simulink model "Task2A"  (R2019b)
settings: Solver=VariableStepAuto  StartTime=0.0  StopTime=10.0  MaxStep=1e-3  RelTol=1e-3
settings Model: Creator=sinow  LastModifiedBy=sinow

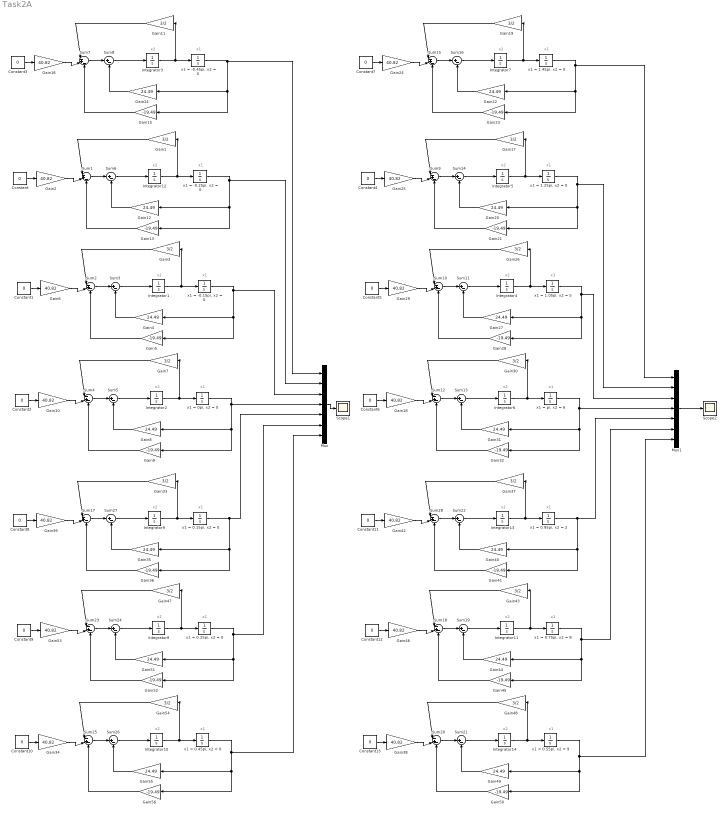
== system Task2A ==
  note: x1
  note: x2
  note: x2
  note: x1
  note: x2
  note: x1
  note: x2
  note: x1
  note: x1
  note: x2
  note: x1
  note: x2
  note: x2
  note: x1
  note: x1
  note: x2
  note: x1
  note: x2
  note: x1
  note: x2
  note: x1
  note: x2
  note: x2
  note: x1
  note: x1
  note: x1
  note: x2
  note: x2
  Constant{,1..13} (14 alike) : Constant  Value=0
  Gain{1,3,7,11,17,19,26,30,33,37,43,47..48,54} (14 alike) : Gain  Gain=3/2
  Gain{2,6,10,16,18,24..25,29,34,38..39,42,46,53} (14 alike) : Gain  Gain=40.82
  Gain{4,8,12,14,20,22,27,31,35,40,44,49,51,55} (14 alike) : Gain  Gain=24.49
  Gain{5,9,13,15,21,23,28,32,36,41,45,50,52,56} (14 alike) : Gain  Gain=-19.49
  Integrator{1..14} (14 alike) : Integrator
  Mux : Mux  Inputs=7
  Mux1 : Mux  Inputs=7
  Scope1 : Scope
  Scope2 : Scope
  Sum{1..2,4,7,9..10,12,15,17..18,20,23,25,28} (14 alike) : Sum  Inputs=|-+-
  Sum{3,5..6,8,11,13..14,16,19,21..22,24,26..27} (14 alike) : Sum  Inputs=|+-
  "x1 = -0.15pi, x2 = 0" : Integrator  InitialCondition=-0.15*pi
  "x1 = -0.25pi, x2 = 0" : Integrator  InitialCondition=-0.25*pi
  "x1 = -0.45pi, x2 = 0" : Integrator  InitialCondition=-0.45*pi
  "x1 = 0.15pi, x2 = 0" : Integrator  InitialCondition=0.15*pi
  "x1 = 0.25pi, x2 = 0" : Integrator  InitialCondition=0.25*pi
  "x1 = 0.45pi, x2 = 0" : Integrator  InitialCondition=0.45*pi
  "x1 = 0.55pi, x2 = 9" : Integrator  InitialCondition=0.55*pi
  "x1 = 0.75pi, x2 = 8" : Integrator  InitialCondition=0.75*pi
  "x1 = 0.95pi, x2 = 2" : Integrator  InitialCondition=0.95*pi
  "x1 = 0pi, x2 = 0" : Integrator
  "x1 = 1.05pi, x2 = 5" : Integrator  InitialCondition=1.05*pi
  "x1 = 1.25pi, x2 = 0" : Integrator  InitialCondition=1.25*pi
  "x1 = 1.45pi, x2 = 0" : Integrator  InitialCondition=1.45*pi
  "x1 = pi, x2 = 6" : Integrator  InitialCondition=pi
  wires:
  Gain13/1 -> Sum1/3
  Integrator12/1 -> Gain1/1, "x1 = -0.25pi, x2 = 0"/1
  Sum6/1 -> Integrator12/1
  Gain12/1 -> Sum6/2
  Gain1/1 -> Sum1/1
  Sum1/1 -> Sum6/1
  Gain2/1 -> Sum1/2
  Constant/1 -> Gain2/1
  Gain5/1 -> Sum2/3
  Sum3/1 -> Integrator1/1
  Integrator1/1 -> Gain3/1, "x1 = -0.15pi, x2 = 0"/1
  Gain4/1 -> Sum3/2
  Gain3/1 -> Sum2/1
  Constant1/1 -> Gain6/1
  Sum2/1 -> Sum3/1
  Gain6/1 -> Sum2/2
  "x1 = 0pi, x2 = 0"/1 -> Mux/4, Gain8/1, Gain9/1
  Gain9/1 -> Sum4/3
  Sum5/1 -> Integrator2/1
  Integrator2/1 -> Gain7/1, "x1 = 0pi, x2 = 0"/1
  Gain8/1 -> Sum5/2
  Gain7/1 -> Sum4/1
  Constant2/1 -> Gain10/1
  Sum4/1 -> Sum5/1
  Gain10/1 -> Sum4/2
  Gain15/1 -> Sum7/3
  Sum8/1 -> Integrator3/1
  Integrator3/1 -> Gain11/1, "x1 = -0.45pi, x2 = 0"/1
  Gain14/1 -> Sum8/2
  Gain11/1 -> Sum7/1
  Constant3/1 -> Gain16/1
  Sum7/1 -> Sum8/1
  Gain16/1 -> Sum7/2
  Sum14/1 -> Integrator5/1
  Integrator5/1 -> Gain17/1, "x1 = 1.25pi, x2 = 0"/1
  Gain20/1 -> Sum14/2
  Gain17/1 -> Sum9/1
  Sum12/1 -> Sum13/1
  Gain30/1 -> Sum12/1
  Constant6/1 -> Gain18/1
  Gain31/1 -> Sum13/2
  Gain18/1 -> Sum12/2
  Gain32/1 -> Sum12/3
  Sum10/1 -> Sum11/1
  Constant5/1 -> Gain29/1
  Integrator4/1 -> Gain26/1, "x1 = 1.05pi, x2 = 5"/1
  Sum11/1 -> Integrator4/1
  Gain25/1 -> Sum9/2
  Sum9/1 -> Sum14/1
  Gain26/1 -> Sum10/1
  Sum16/1 -> Integrator7/1
  Gain24/1 -> Sum15/2
  Integrator6/1 -> Gain30/1, "x1 = pi, x2 = 6"/1
  Gain22/1 -> Sum16/2
  Constant7/1 -> Gain24/1
  Gain19/1 -> Sum15/1
  Integrator7/1 -> Gain19/1, "x1 = 1.45pi, x2 = 0"/1
  Constant4/1 -> Gain25/1
  Sum15/1 -> Sum16/1
  Gain27/1 -> Sum11/2
  Sum13/1 -> Integrator6/1
  Gain29/1 -> Sum10/2
  Gain23/1 -> Sum15/3
  Gain28/1 -> Sum10/3
  Gain21/1 -> Sum9/3
  Gain36/1 -> Sum17/3
  Sum27/1 -> Integrator9/1
  Integrator9/1 -> Gain33/1, "x1 = 0.15pi, x2 = 0"/1
  Gain35/1 -> Sum27/2
  Gain33/1 -> Sum17/1
  Gain45/1 -> Sum18/3
  Gain41/1 -> Sum28/3
  Gain44/1 -> Sum19/2
  Constant11/1 -> Gain42/1
  Sum28/1 -> Sum22/1
  Gain43/1 -> Sum18/1
  Integrator11/1 -> Gain43/1, "x1 = 0.75pi, x2 = 8"/1
  Constant12/1 -> Gain46/1
  Sum18/1 -> Sum19/1
  Gain50/1 -> Sum20/3
  Integrator14/1 -> Gain48/1, "x1 = 0.55pi, x2 = 9"/1
  Gain40/1 -> Sum22/2
  Gain38/1 -> Sum20/2
  Gain48/1 -> Sum20/1
  Sum20/1 -> Sum21/1
  Gain49/1 -> Sum21/2
  Integrator13/1 -> Gain37/1, "x1 = 0.95pi, x2 = 2"/1
  Sum25/1 -> Sum26/1
  Sum21/1 -> Integrator14/1
  Gain54/1 -> Sum25/1
  Constant10/1 -> Gain34/1
  Gain55/1 -> Sum26/2
  Gain34/1 -> Sum25/2
  Gain56/1 -> Sum25/3
  Integrator10/1 -> Gain54/1, "x1 = 0.45pi, x2 = 0"/1
  Gain37/1 -> Sum28/1
  Sum26/1 -> Integrator10/1
  Gain46/1 -> Sum18/2
  Gain53/1 -> Sum23/2
  Sum23/1 -> Sum24/1
  Constant9/1 -> Gain53/1
  Integrator8/1 -> Gain47/1, "x1 = 0.25pi, x2 = 0"/1
  Gain52/1 -> Sum23/3
  Sum19/1 -> Integrator11/1
  Sum24/1 -> Integrator8/1
  Gain42/1 -> Sum28/2
  Gain51/1 -> Sum24/2
  Constant13/1 -> Gain38/1
  Sum22/1 -> Integrator13/1
  Constant8/1 -> Gain39/1
  Sum17/1 -> Sum27/1
  Gain47/1 -> Sum23/1
  Gain39/1 -> Sum17/2
  Mux/1 -> Scope1/1
  "x1 = -0.45pi, x2 = 0"/1 -> Mux/1, Gain14/1, Gain15/1
  "x1 = -0.25pi, x2 = 0"/1 -> Mux/2, Gain12/1, Gain13/1
  "x1 = -0.15pi, x2 = 0"/1 -> Mux/3, Gain4/1, Gain5/1
  "x1 = 0.15pi, x2 = 0"/1 -> Gain35/1, Gain36/1, Mux/5
  "x1 = 0.25pi, x2 = 0"/1 -> Mux/6, Gain51/1, Gain52/1
  "x1 = 0.45pi, x2 = 0"/1 -> Mux/7, Gain55/1, Gain56/1
  "x1 = 0.55pi, x2 = 9"/1 -> Mux1/7, Gain49/1, Gain50/1
  Mux1/1 -> Scope2/1
  "x1 = 0.75pi, x2 = 8"/1 -> Gain44/1, Gain45/1, Mux1/6
  "x1 = 1.25pi, x2 = 0"/1 -> Mux1/2, Gain20/1, Gain21/1
  "x1 = 1.05pi, x2 = 5"/1 -> Mux1/3, Gain27/1, Gain28/1
  "x1 = pi, x2 = 6"/1 -> Mux1/4, Gain31/1, Gain32/1
  "x1 = 1.45pi, x2 = 0"/1 -> Mux1/1, Gain22/1, Gain23/1
  "x1 = 0.95pi, x2 = 2"/1 -> Gain40/1, Gain41/1, Mux1/5
